simulink model "nodo_posicion_velocidad"  (R2017a)
settings: Solver=FixedStepAuto  StartTime=0.0  StopTime=10.0  RelTol=1e-3
undefined symbols (not defined in the file): Angular, Linear, Orientation, Position
libraries: robotlib x5
settings Model: Creator=dani  LastModifiedBy=dani
settings OptimizationCC: PassReuseOutputArgsAs=Individual arguments  MaxStackSize=64
settings DebuggingCC: ParameterTunabilityLossMsg=error
settings HardwareCC: ProdBitPerPointer=32  ProdBitPerSizeT=32  ProdBitPerPtrDiffT=32  ProdLargestAtomicInteger=Long  ProdLargestAtomicFloat=Double  ProdWordSize=32  ProdHWDeviceType=ARM Compatible->ARM Cortex  UseEmbeddedCoderFeatures=off
settings SFSimCC: MATLABDynamicMemAlloc=off
settings RTWCC: SystemTargetFile=ert.tlc  HardwareBoard=Robot Operating System (ROS)  TLCOptions="-aInlineSetEventsForThisBaseRateFcn=TLC_FALSE -aSuppressMultiTaskScheduler=TLC_FALSE  -aRateBasedStepFcn=0"  TemplateMakefile=ert_default_tmf  Description=Embedded Coder  GenerateReport=on  Toolchain=Catkin  IncludeHyperlinkInReport=on  LaunchReport=on  TargetLang=C++  GenerateTraceInfo=on  GenerateTraceReport=on  GenerateTraceReportSl=on  GenerateTraceReportSf=on  GenerateTraceReportEml=on
settings CodeAppCC: ForceParamTrailComments=on  IgnoreCustomStorageClasses=off  OperatorAnnotations=on  SimulinkDataObjDesc=on  SFDataObjDesc=on  MATLABFcnDesc=on  InsertBlockDesc=on  MATLABSourceComments=on
settings ERTTargetCC: SupportNonInlinedSFcns=on

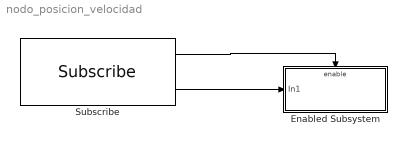
== system nodo_posicion_velocidad ==
  Enabled Subsystem : Subsystem  TreatAsAtomicUnit=on
  Subscribe : robotlib/Subscribe  SourceLibraryInfo=This block requires Robotics System Toolbox  topicSource=Specify your own  topic=/vehicle_speed  messageType=geometry_msgs/Twist  sampleTime=-1  messageQueueLength=1
      settings: SourceProductBaseCode=RO
  wires:
  Subscribe/2 -> Enabled Subsystem/1(In1)
  Subscribe/1 -> Enabled Subsystem/Enable

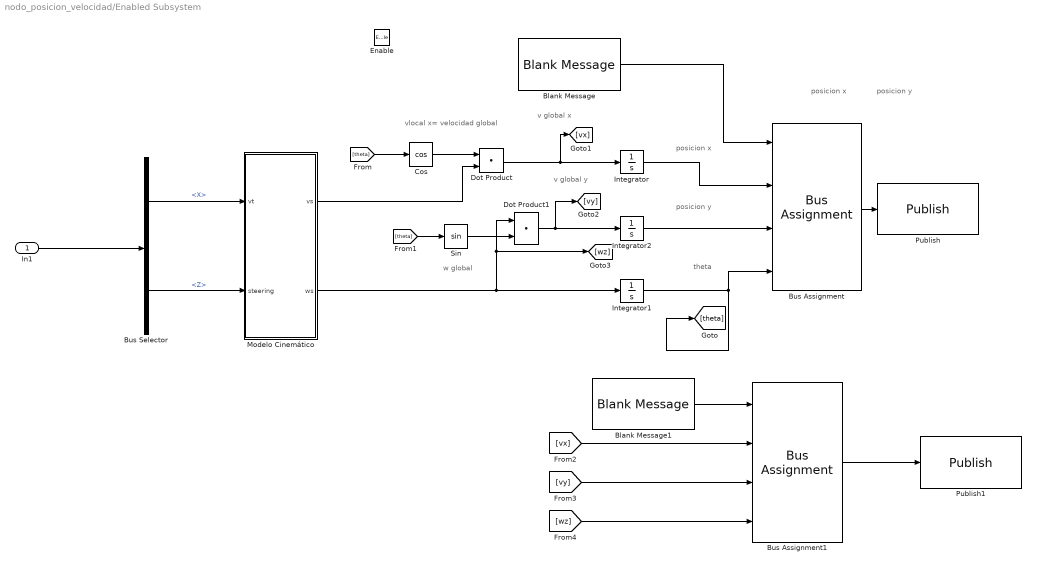
== system nodo_posicion_velocidad/Enabled Subsystem ==
  note: w global
  note: posicion x
  note: posicion y
  note: v global y
  note: v global x
  note: posicion y
  note: posicion x
  note: theta
  note: vlocal x= velocidad global
  In1 : Inport
  Enable : EnablePort
  Blank Message : robotlib/Blank Message  SourceLibraryInfo=This block requires Robotics System Toolbox  messageType=geometry_msgs/Pose  SampleTime=inf
      settings: SourceProductBaseCode=RO
  Blank Message1 : robotlib/Blank Message  SourceLibraryInfo=This block requires Robotics System Toolbox  messageType=geometry_msgs/Twist  SampleTime=inf
      settings: SourceProductBaseCode=RO
  Bus Assignment : BusAssignment  AssignedSignals=Position.X,Position.Y,Orientation.Z
  Bus Assignment1 : BusAssignment  AssignedSignals=Linear.X,Linear.Y,Angular.Z
  Bus Selector : BusSelector  OutputSignals=Linear.X,Angular.Z
  Cos : Trigonometry  Operator=cos
  Dot Product : DotProduct  InputSameDT=on  OutDataTypeStr=Inherit: Inherit via internal rule
  Dot Product1 : DotProduct  InputSameDT=on  OutDataTypeStr=Inherit: Inherit via internal rule
  Integrator : Integrator
  Integrator1 : Integrator
  Integrator2 : Integrator
  Modelo Cinemático : Subsystem
  Publish : robotlib/Publish  SourceLibraryInfo=This block requires Robotics System Toolbox  topicSource=Specify your own  topic=/posicion  messageType=geometry_msgs/Pose  messageQueueLength=1
      settings: SourceProductBaseCode=RO
  Publish1 : robotlib/Publish  SourceLibraryInfo=This block requires Robotics System Toolbox  topicSource=Specify your own  topic=/velocity  messageType=geometry_msgs/Twist  messageQueueLength=1
      settings: SourceProductBaseCode=RO
  Sin : Trigonometry
  wires:
  In1/1 -> Bus Selector/1
  Integrator1/1 -> Bus Assignment/4, [theta]
  Cos/1 -> Dot Product/1
  [theta] -> Cos/1
  [theta] -> Sin/1
  Sin/1 -> Dot Product1/2
  Dot Product/1 -> [vx], Integrator/1
  Dot Product1/1 -> Integrator2/1, [vy]
  Blank Message/1 -> Bus Assignment/1
  Integrator/1 -> Bus Assignment/2
  Integrator2/1 -> Bus Assignment/3
  Bus Assignment/1 -> Publish/1
  Blank Message1/1 -> Bus Assignment1/1
  [vx] -> Bus Assignment1/2
  [vy] -> Bus Assignment1/3
  [wz] -> Bus Assignment1/4
  Bus Assignment1/1 -> Publish1/1
  Bus Selector/1 -> Modelo Cinemático/1(vt)  "<X>"
  Bus Selector/2 -> Modelo Cinemático/2(steering)  "<Z>"
  Modelo Cinemático/1(vs) -> Dot Product/2
  Modelo Cinemático/2(ws) -> Integrator1/1, [wz], Dot Product1/1

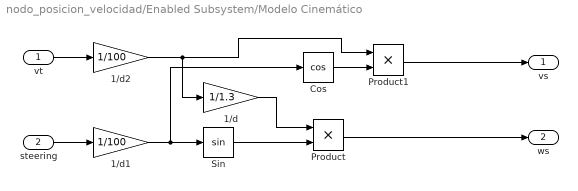
== system nodo_posicion_velocidad/Enabled Subsystem/Modelo Cinemático ==
  vt : Inport
  steering : Inport  Port=2
  1/d : Gain  Gain=1/1.3
  1/d1 : Gain  Gain=1/100
  1/d2 : Gain  Gain=1/100
  Cos : Trigonometry  Operator=cos
  Product : Product
  Product1 : Product
  Sin : Trigonometry
  vs : Outport
  ws : Outport  Port=2
  wires:
  1/d1/1 -> Cos/1, Sin/1
  steering/1 -> 1/d1/1
  vt/1 -> 1/d2/1
  Cos/1 -> Product1/2
  Sin/1 -> Product/2
  Product1/1 -> vs/1
  Product/1 -> ws/1
  1/d/1 -> Product/1
  1/d2/1 -> 1/d/1, Product1/1
